simulink model "Control_BC_ACT"  (R2023b)
settings: Solver=VariableStepAuto  StartTime=0.0  StopTime=10.0  RelTol=1e-3
settings Model: Creator=Alberto  LastModifiedBy=Alberto

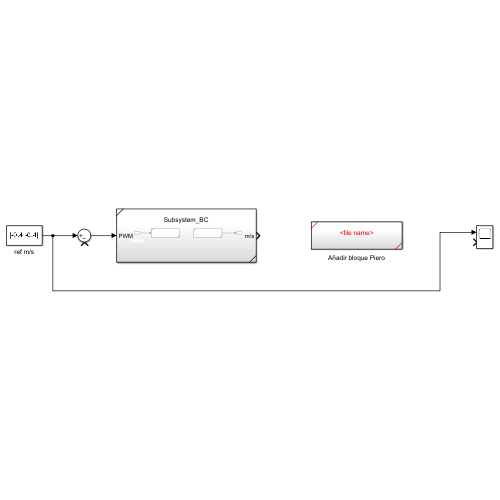
[thumbnail: Simulink's stored preview of the top-level diagram]
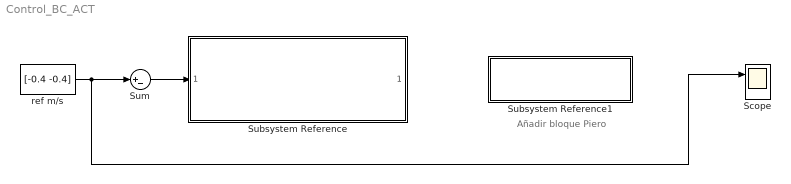
== system Control_BC_ACT ==
  note: Añadir bloque Piero
  Scope : Scope  NumInputPorts=2
  Subsystem Reference : Subsystem  ReferencedSubsystem=Subsystem_BC
  Subsystem Reference1 : Subsystem  ReferencedSubsystem=<file name>
  Sum : Sum  Inputs=|+-
  ref m/s : Constant  Value=[-0.4 -0.4]
  wires:
  ref m/s/1 -> Scope/1, Sum/1
  Sum/1 -> Subsystem Reference/1

== system Control_BC_ACT/Subsystem Reference1 ==
